simulink model "WPT_closedloop"  (R2016a)
settings: Solver=ode23tb  StartTime=0.0  StopTime=0.1  RelTol=1e-3
libraries: powerlib x22, powerlib_meascontrol x2, simulink x1
settings Model: Creator=linxing  LastModifiedBy=linxing

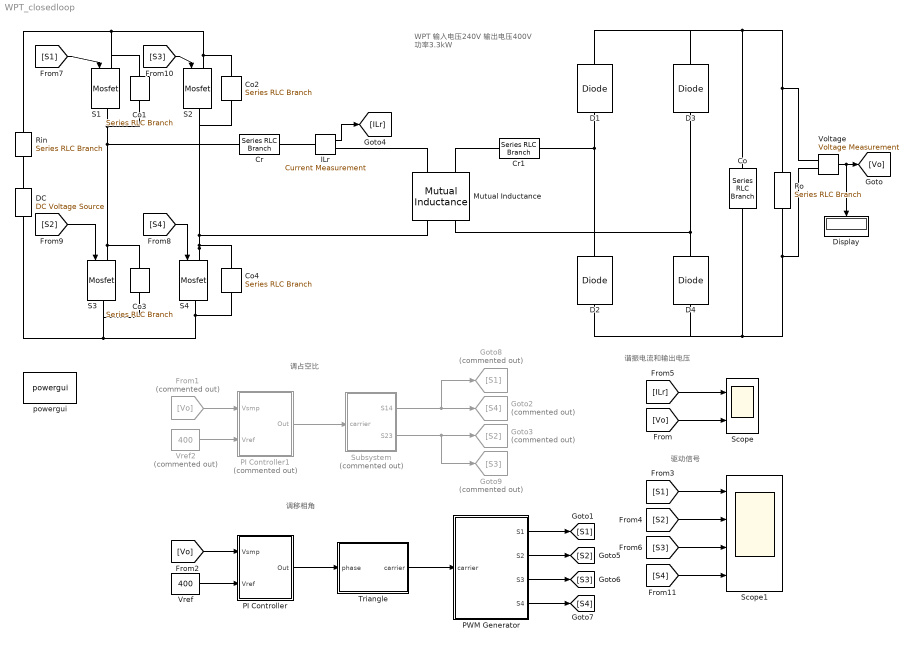
== system WPT_closedloop ==
  note: 谐振电流和输出电压
  note: 驱动信号
  note: WPT
      | 输入电压240V
      | 输出电压400V
      | 功率3.3kW
  note: 调占空比
  note: 调移相角
  Co : powerlib/Elements/Series RLC Branch  LConnTagsString=__new0  RConnTagsString=__new0  BranchType=RC  Resistance=0.001  Inductance=43.48e-6  SetiL0=off  InitialCurrent=0  Capacitance=220e-6  Setx0=off  InitialVoltage=0  Measurements=None
  Co{1..4} (4 alike) : powerlib/Elements/Series RLC Branch  LConnTagsString=__new0  RConnTagsString=__new0  BranchType=C  Resistance=0.001  Inductance=43.48e-6  SetiL0=off  InitialCurrent=0  Capacitance=90e-12  Setx0=off  InitialVoltage=0  Measurements=None
  Cr : powerlib/Elements/Series RLC Branch  LConnTagsString=__new0  RConnTagsString=__new0  BranchType=C  Resistance=1  Inductance=43.48e-6  SetiL0=off  InitialCurrent=0  Capacitance=39.8e-9  Setx0=off  InitialVoltage=0  Measurements=None
  Cr1 : powerlib/Elements/Series RLC Branch  LConnTagsString=__new0  RConnTagsString=__new0  BranchType=C  Resistance=1  Inductance=43.48e-6  SetiL0=off  InitialCurrent=0  Capacitance=27.8e-9  Setx0=off  InitialVoltage=0  Measurements=None
  D{1..4} (4 alike) : powerlib/Power Electronics/Diode  Ron=0.001  Lon=0  Vf=0.8  IC=0  UseSnubber=off  Rs=500  Cs=250e-9  Measurements=off
  DC : powerlib/Electrical Sources/DC Voltage Source  Amplitude=240  Measurements=None
  Display : Display
  From1 : From  Commented=on  GotoTag=Vo
  Goto2 : Goto  Commented=on  GotoTag=S4
  Goto3 : Goto  Commented=on  GotoTag=S2
  Goto8 : Goto  Commented=on  GotoTag=S1
  Goto9 : Goto  Commented=on  GotoTag=S3
  ILr : powerlib/Measurements/Current Measurement  PhasorSimulation=off  OutputType=Complex  PSBequivalent=0
  Mutual Inductance : powerlib/Elements/Mutual Inductance  LConnTagsString=a|b  RConnTagsString=A|B  TypeOfMutual=Two or three windings with equal mutual terms  NumberOfWindings=3  SelfImpedance1=[.01 8.793e-05]  SelfImpedance2=[ .01 1.261e-04]  ThreeWindings=off  SelfImpedance3=[ 1.1 1.1e-03]  MutualImpedance=[0.1 2.106e-05]  InductanceMatrix="[1.0 0.9  0.9 ;  0.9 1.0  0.9;  0.9 0.9 1.0 ] * 1e-3"  ResistanceMatrix="[1.0 0.9  0.9 ;  0.9 1.0  0.9;  0.9 0.9 1.0 ]"  Measurements=None
      settings: AttributesFormatString=\n
  PI Controller : Subsystem
  PI Controller1 : Subsystem  Commented=on
  PWM Generator : Subsystem
  Rin : powerlib/Elements/Series RLC Branch  LConnTagsString=__new0  RConnTagsString=__new0  BranchType=R  Resistance=0.001  Inductance=43.48e-6  SetiL0=off  InitialCurrent=0  Capacitance=233e-9  Setx0=off  InitialVoltage=0  Measurements=None
  Ro : powerlib/Elements/Series RLC Branch  LConnTagsString=__new0  RConnTagsString=__new0  BranchType=R  Resistance=50  Inductance=43.48e-6  SetiL0=off  InitialCurrent=0  Capacitance=100e-6  Setx0=off  InitialVoltage=0  Measurements=None
  S{1..4} (4 alike) : powerlib/Power Electronics/Mosfet  Ron=0.1  Lon=0  Rd=0.01  Vfd=0  IC=0  Rs=1e5  Cs=inf  Measurements=off
  Scope : Scope  NumInputPorts=2
  Scope1 : Scope  NumInputPorts=4
  Subsystem : Subsystem  Commented=on
  Triangle : Subsystem  mask{f=85000}
      mask prompts: f "Frequency"
  Voltage : powerlib/Measurements/Voltage Measurement  PhasorSimulation=off  OutputType=Complex  PSBequivalent=0
  Vref : Constant  Value=400
  Vref2 : Constant  Commented=on  Value=400
  powergui : powerlib/powergui  Priority=1  SimulationMode=Discrete  SolverType=Tustin/Backward Euler (TBE)  SampleTime=50e-9  frequency=60  SPID=off  DisableSnubberDevices=off  DisableRonSwitches=off  DisableVfSwitches=off  SwTol=0  DisplayEquations=off  Interpol=off  ExternalGateDelay=off  methode=off  Ts=10  FunctionMessages=off  echomessages=off  HookPort=off  EnableUseOfTLC=off  x0status=blocks  frequencyindice=0  Pbase=100e6  ErrMax=1e-4  Iterations=50  UnitsV=kV  UnitsW=MW  buscounter=0  RestoreLinks=warning  ResistiveCurrentMeasurement=off  Frange=[0:2:500]  Ylog=off  Xlog=on  ShowGrid=off  save=off  variable=ZData  structure=0  ZoomFFT=off  StartTime=0.0  cycles=1  DisplayStyle=1  fundamental=60  FreqAxis=off  MaxFrequency=1000  frequencyindicesteady=1  RmsSteady=1  display=off
  wires:
  Voltage/1 -> Display/1, [Vo]
  Subsystem/1(S14) -> Goto8/1, Goto2/1
  [Vo] -> PI Controller/1(Vsmp)
  Vref/1 -> PI Controller/2(Vref)
  ILr/1 -> [ILr]
  [S1] -> S1/1
  [S4] -> S4/1
  [S2] -> S3/1
  [S3] -> S2/1
  [ILr] -> Scope/1
  [Vo] -> Scope/2
  Triangle/1(carrier) -> PWM Generator/1(carrier)
  PWM Generator/1(S1) -> [S1]
  PWM Generator/2(S2) -> [S2]
  PWM Generator/3(S3) -> [S3]
  PWM Generator/4(S4) -> [S4]
  From1/1 -> PI Controller1/1(Vsmp)
  Vref2/1 -> PI Controller1/2(Vref)
  Subsystem/2(S23) -> Goto3/1, Goto9/1
  [S1] -> Scope1/1
  [S2] -> Scope1/2
  [S3] -> Scope1/3
  [S4] -> Scope1/4
  PI Controller1/1(Out) -> Subsystem/1(carrier)
  PI Controller/1(Out) -> Triangle/1(phase)
  connections:
  Ro/LConn1 -- Voltage/LConn1 -- D3/RConn1 -- D1/RConn1 -- Co/LConn1
  Ro/RConn1 -- Voltage/LConn2 -- D4/LConn1 -- D2/LConn1 -- Co/RConn1
  DC/RConn1 -- Rin/RConn1
  ILr/LConn1 -- Cr/RConn1
  D1/LConn1 -- Cr1/RConn1 -- D2/RConn1
  D3/LConn1 -- Mutual Inductance/RConn2 -- D4/RConn1
  Rin/LConn1 -- Co1/LConn1 -- S1/LConn1 -- Co2/LConn1 -- S2/LConn1
  S1/RConn1 -- Co1/RConn1 -- Cr/LConn1 -- Co3/LConn1 -- S3/LConn1
  S4/LConn1 -- Co2/RConn1 -- S2/RConn1 -- Mutual Inductance/RConn1 -- Co4/LConn1
  S4/RConn1 -- Co4/RConn1 -- Co3/RConn1 -- S3/RConn1 -- DC/LConn1
  Mutual Inductance/LConn1 -- ILr/RConn1
  Mutual Inductance/LConn2 -- Cr1/LConn1

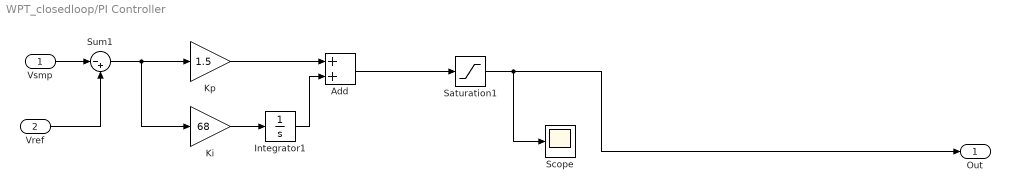
== system WPT_closedloop/PI Controller ==
  Vsmp : Inport
  Vref : Inport  Port=2
  Add : Sum
  Integrator1 : Integrator
  Ki : Gain  Gain=68
  Kp : Gain  Gain=1.5
  Saturation1 : Saturate  UpperLimit=180  LowerLimit=0
  Scope : Scope
  Sum1 : Sum  Inputs=|-+
  Out : Outport
  wires:
  Saturation1/1 -> Scope/1, Out/1
  Vsmp/1 -> Sum1/1
  Kp/1 -> Add/1
  Integrator1/1 -> Add/2
  Ki/1 -> Integrator1/1
  Sum1/1 -> Ki/1, Kp/1
  Vref/1 -> Sum1/2
  Add/1 -> Saturation1/1

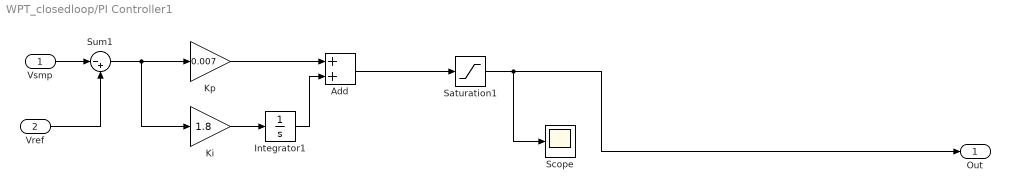
== system WPT_closedloop/PI Controller1 ==
  Vsmp : Inport
  Vref : Inport  Port=2
  Add : Sum
  Integrator1 : Integrator
  Ki : Gain  Gain=1.8
  Kp : Gain  Gain=0.007
  Saturation1 : Saturate  LowerLimit=0.01
  Scope : Scope
  Sum1 : Sum  Inputs=|-+
  Out : Outport
  wires:
  Add/1 -> Saturation1/1
  Vref/1 -> Sum1/2
  Sum1/1 -> Kp/1, Ki/1
  Ki/1 -> Integrator1/1
  Integrator1/1 -> Add/2
  Kp/1 -> Add/1
  Vsmp/1 -> Sum1/1
  Saturation1/1 -> Out/1, Scope/1

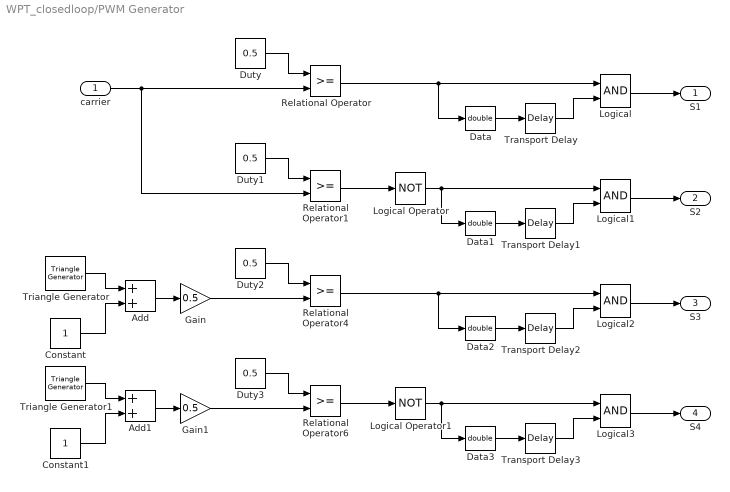
== system WPT_closedloop/PWM Generator ==
  carrier : Inport
  Add : Sum
  Add1 : Sum
  Constant : Constant
  Constant1 : Constant
  Data{,1..3} (4 alike) : DataTypeConversion  OutDataTypeStr=double
  Duty{,1..3} (4 alike) : Constant  Value=0.5
  Gain : Gain  Gain=0.5
  Gain1 : Gain  Gain=0.5
  Logical{,1..3} (4 alike) : Logic  AllPortsSameDT=off  OutDataTypeStr=boolean
  Logical Operator : Logic  Operator=NOT  AllPortsSameDT=off  OutDataTypeStr=boolean
  Logical Operator1 : Logic  Operator=NOT  AllPortsSameDT=off  OutDataTypeStr=boolean
  Relational Operator{,1,4,6} (4 alike) : RelationalOperator  OutDataTypeStr=boolean
  Transport Delay{,1..3} (4 alike) : TransportDelay  DelayTime=100e-9
  Triangle Generator : powerlib_meascontrol/Pulse & Signal Generators/Triangle Generator  Freq=85e3  Phase=0  Ts=0
  Triangle Generator1 : powerlib_meascontrol/Pulse & Signal Generators/Triangle Generator  Freq=85e3  Phase=0  Ts=0
  S1 : Outport
  S2 : Outport  Port=2
  S3 : Outport  Port=3
  S4 : Outport  Port=4
  wires:
  Duty/1 -> Relational Operator/1
  Transport Delay2/1 -> Logical2/2
  Relational Operator4/1 -> Logical2/1, Data2/1
  Duty2/1 -> Relational Operator4/1
  Constant1/1 -> Add1/2
  Triangle Generator1/1 -> Add1/1
  Add1/1 -> Gain1/1
  Gain1/1 -> Relational Operator6/2
  Add/1 -> Gain/1
  Gain/1 -> Relational Operator4/2
  Constant/1 -> Add/2
  Triangle Generator/1 -> Add/1
  Relational Operator/1 -> Logical/1, Data/1
  Duty3/1 -> Relational Operator6/1
  Logical Operator1/1 -> Logical3/1, Data3/1
  Relational Operator6/1 -> Logical Operator1/1
  Transport Delay3/1 -> Logical3/2
  Relational Operator1/1 -> Logical Operator/1
  Duty1/1 -> Relational Operator1/1
  Transport Delay/1 -> Logical/2
  carrier/1 -> Relational Operator1/2, Relational Operator/2
  Logical Operator/1 -> Logical1/1, Data1/1
  Transport Delay1/1 -> Logical1/2
  Data/1 -> Transport Delay/1
  Data1/1 -> Transport Delay1/1
  Data2/1 -> Transport Delay2/1
  Data3/1 -> Transport Delay3/1
  Logical/1 -> S1/1
  Logical1/1 -> S2/1
  Logical2/1 -> S3/1
  Logical3/1 -> S4/1

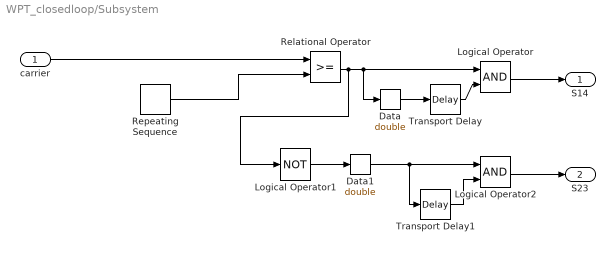
== system WPT_closedloop/Subsystem ==
  carrier : Inport
  Data : DataTypeConversion  OutDataTypeStr=double
  Data1 : DataTypeConversion  OutDataTypeStr=double
  Logical Operator : Logic  AllPortsSameDT=off  OutDataTypeStr=boolean
  Logical Operator1 : Logic  Operator=NOT  AllPortsSameDT=off  OutDataTypeStr=boolean
  Logical Operator2 : Logic  AllPortsSameDT=off  OutDataTypeStr=boolean
  Relational Operator : RelationalOperator  OutDataTypeStr=boolean
  Repeating Sequence : simulink/Sources/Repeating Sequence  rep_seq_t=[0 1/85e3]  rep_seq_y=[0 1]
  Transport Delay : TransportDelay  DelayTime=200e-9
  Transport Delay1 : TransportDelay  DelayTime=200e-9
  S14 : Outport
  S23 : Outport  Port=2
  wires:
  Logical Operator/1 -> S14/1
  Transport Delay1/1 -> Logical Operator2/2
  Logical Operator1/1 -> Data1/1
  Transport Delay/1 -> Logical Operator/2
  Relational Operator/1 -> Data/1, Logical Operator/1, Logical Operator1/1
  Logical Operator2/1 -> S23/1
  Data1/1 -> Transport Delay1/1, Logical Operator2/1
  Data/1 -> Transport Delay/1
  carrier/1 -> Relational Operator/1
  Repeating Sequence/1 -> Relational Operator/2

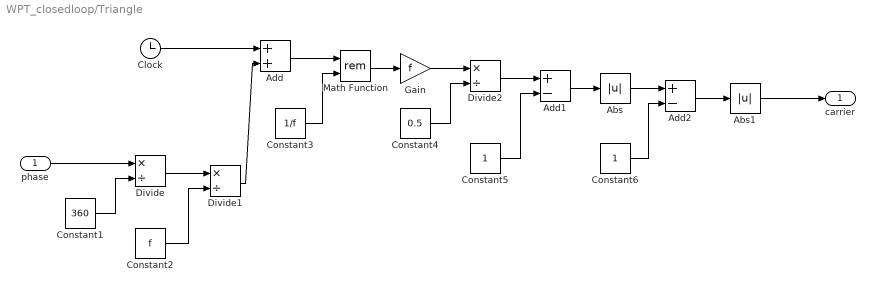
== system WPT_closedloop/Triangle ==
  phase : Inport
  Abs : Abs
  Abs1 : Abs
  Add : Sum
  Add1 : Sum  Inputs=+-
  Add2 : Sum  Inputs=+-
  Clock : Clock
  Constant1 : Constant  Value=360
  Constant2 : Constant  Value=f  SampleTime=1e-6
  Constant3 : Constant  Value=1/f  SampleTime=1e-6
  Constant4 : Constant  Value=0.5
  Constant5 : Constant
  Constant6 : Constant
  Divide : Product  Inputs=*/
  Divide1 : Product  Inputs=*/
  Divide2 : Product  Inputs=*/
  Gain : Gain  Gain=f
  Math Function : Math  Operator=rem  SaturateOnIntegerOverflow=on
  carrier : Outport
  wires:
  phase/1 -> Divide/1
  Add1/1 -> Abs/1
  Divide1/1 -> Add/2
  Constant1/1 -> Divide/2
  Divide/1 -> Divide1/1
  Constant4/1 -> Divide2/2
  Constant5/1 -> Add1/2
  Constant6/1 -> Add2/2
  Add2/1 -> Abs1/1
  Math Function/1 -> Gain/1
  Clock/1 -> Add/1
  Gain/1 -> Divide2/1
  Abs/1 -> Add2/1
  Divide2/1 -> Add1/1
  Constant2/1 -> Divide1/2
  Abs1/1 -> carrier/1
  Add/1 -> Math Function/1
  Constant3/1 -> Math Function/2
